simulink model "SimulinkModel"  (R2023a)
settings: Solver=FixedStepAuto  StartTime=0.0  StopTime=10  FixedStep=DT  RelTol=1e-3
values from neighbouring files (symbols this model uses):
  A = [0 1 0 0 ... (first row only)    [Main.m]
  AO = A-KO*C    [Main.m]
  B1 = [0; b12; 0; b14]    [Main.m]
  B2 = [0 0 0 0 ... (first row only)    [Main.m]
  BO = B1-KO*D1    [Main.m]
  C = [1 0 0 0 ... (first row only)    [Main.m]
  Ce = [ 1 0 0 0]    [Main.m]
  Ceps = [-ks/ms -bs/ms 0 0 0 ... (first row only)    [Main.m]
  CO = eye(n)    [Main.m]
  D1 = [0; 1/ms]    [Main.m]
  D2 = [0 1 0 0 ... (first row only)    [Main.m]
  De1 = 0    [Main.m]
  De2 = [0 0 1 -1]    [Main.m]
  Deps = [1/ms; 0; 0; 0;0; 0]    [Main.m]
  DT = 1e-3    (= 0.001)    [Main.m]
  e0 = x0(1)-r0    [Main.m]
  KI = K(:,n+1:n+m)    [Main.m]
  KO = Km.'    [Main.m]
  KS = K(:,1:n)    [Main.m]
  m = 1    [Main.m]
  n = size(V)    [JCF.m]    (also in Main.m = 4)
  p = 1    [Main.m]
  PLANT = 1    [Main.m]
  q = length(index{i})    [JCF.m]    (also in Main.m = 2)
  r = w(4)    [F.m]    (also in Main.m = 4; reference.m = 0.34671875)
  r0 = ells-g*ms/ks    (= 0.367749146758)    [Main.m]    (also in reference.m = 0.34671875)
  tilde_x_init = x_init-x0    [Main.m]
  u0 = 0    [Main.m]
  v = 10    [Main.m]
  w0 = [d0; nu0; r0]    [Main.m]
  x0 = [ells-g*ms/ks ... (first row only)    [Main.m]
  x_init = [zs_init-zu_init ... (first row only)    [Main.m]
  xO_init = tilde_x_init    [Main.m]
  y0 = [x0(1) ... (first row only)    [Main.m]
libraries: simulink x3
settings Model: Creator=nicola.mimmo2  LastModifiedBy=loreb
settings DebuggingCC: UnconnectedInputMsg=warning  UnconnectedOutputMsg=warning  UnconnectedLineMsg=warning
settings ModelReferenceCC: EnableRefExpFcnMdlSchedulingChecks=on
settings RTWCC: DLArmComputeVersion=19.05

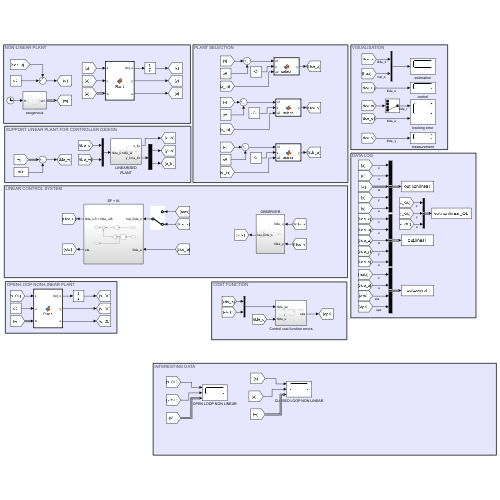
[thumbnail: Simulink's stored preview of the top-level diagram]
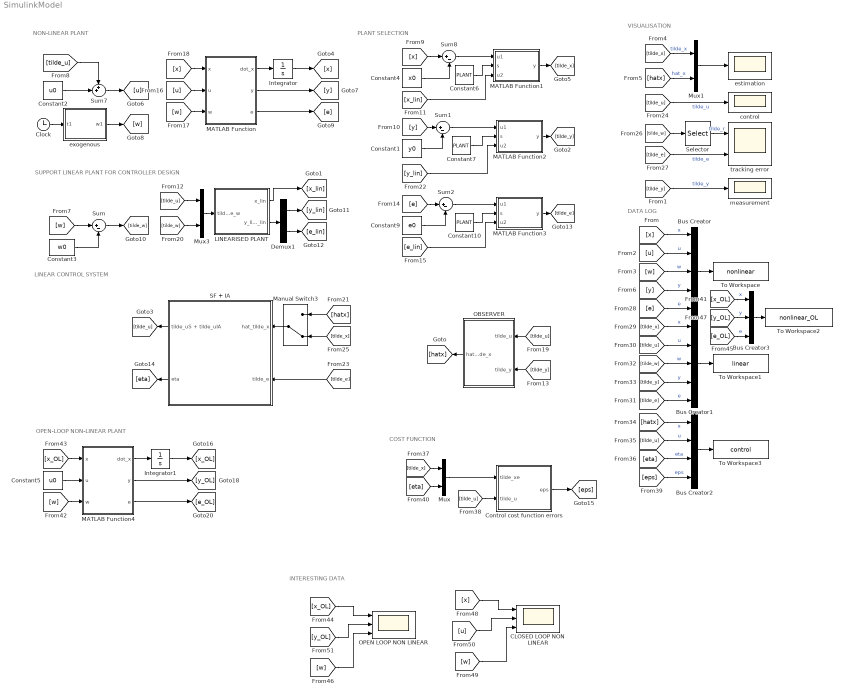
== system SimulinkModel ==
  note: DATA LOG
  note: VISUALISATION
  note: PLANT SELECTION
  note: NON-LINEAR PLANT
  note: SUPPORT LINEAR PLANT FOR CONTROLLER DESIGN
  note: LINEAR CONTROL SYSTEM
  note: OPEN-LOOP NON-LINEAR PLANT
  note: COST FUNCTION
  note: iNTERESTING DATA
  Bus Creator : BusCreator  Inputs=5
  Bus Creator1 : BusCreator  Inputs=5
  Bus Creator2 : BusCreator  Inputs=4
  Bus Creator3 : BusCreator  Inputs=3
  CLOSED LOOP NON LINEAR : Scope  NumInputPorts=3
  Clock : Clock
  Constant1 : Constant  Value=y0
  Constant10 : Constant  Value=PLANT
  Constant2 : Constant  Value=u0
  Constant3 : Constant  Value=w0
  Constant4 : Constant  Value=x0
  Constant5 : Constant  Value=u0
  Constant6 : Constant  Value=PLANT
  Constant7 : Constant  Value=PLANT
  Constant9 : Constant  Value=e0
  Control cost function errors : Subsystem
  Demux1 : Demux  Outputs=[q m]
  Integrator : Integrator  InitialCondition=x_init
  Integrator1 : Integrator  InitialCondition=x_init
  LINEARISED PLANT : Subsystem
  MATLAB Function : MATLAB Function  TreatAsAtomicUnit=on
  MATLAB Function1 : MATLAB Function  TreatAsAtomicUnit=on
  MATLAB Function2 : MATLAB Function  TreatAsAtomicUnit=on
  MATLAB Function3 : MATLAB Function  TreatAsAtomicUnit=on
  MATLAB Function4 : MATLAB Function  TreatAsAtomicUnit=on
  Manual Switch3 : ManualSwitch  CurrentSetting=0
  Mux : Mux  Inputs=2
  Mux1 : Mux  Inputs=2
  Mux3 : Mux  Inputs=2
  OBSERVER : Subsystem
  OPEN LOOP NON LINEAR : Scope  NumInputPorts=3
  SF + IA : Subsystem
  Selector : Selector  InputPortWidth=r  IndexOptions=Index vector (dialog)  Indices=[r-m+1:1:r]  OutputSizes=1
  Sum{,1..2,8} (4 alike) : Sum  Inputs=|+-
  Sum7 : Sum  Inputs=++|
  To Workspace : ToWorkspace  VariableName=nonlinear  SaveFormat=Timeseries  SampleTime=-1
  To Workspace1 : ToWorkspace  VariableName=linear  SaveFormat=Timeseries  SampleTime=-1
  To Workspace2 : ToWorkspace  VariableName=nonlinear_OL  SaveFormat=Timeseries  SampleTime=-1
  To Workspace3 : ToWorkspace  VariableName=control  SaveFormat=Timeseries  SampleTime=-1
  control : Scope
  estimation : Scope
  exogenous : Subsystem
  measurement : Scope
  tracking error : Scope  NumInputPorts=2
  wires:
  Integrator/1 -> [x]
  Constant3/1 -> Sum/2
  Mux3/1 -> LINEARISED PLANT/1(tilde_u tilde_w)
  OBSERVER/1(hat_tilde_x) -> [hatx]
  [tilde_x] -> Mux1/1  "tilde_x"
  [hatx] -> Mux1/2  "hat_x"
  SF + IA/1(tilde_uS + tilde_uIA) -> [tilde_u]
  Constant2/1 -> Sum7/2
  Sum7/1 -> [u]
  [tilde_u] -> Sum7/1
  Constant1/1 -> Sum1/2
  Sum1/1 -> MATLAB Function2/1(u1)
  [y] -> Sum1/1
  [w] -> Sum/1
  [x] -> Sum8/1
  Constant4/1 -> Sum8/2
  Sum8/1 -> MATLAB Function1/1(u1)
  [x_lin] -> MATLAB Function1/3(u2)
  [tilde_e] -> SF + IA/2(tilde_e)
  [tilde_u] -> Mux3/1
  [u] -> MATLAB Function/2(u)
  [w] -> MATLAB Function/3(w)
  [x] -> MATLAB Function/1(x)
  Sum/1 -> [tilde_w]
  [tilde_w] -> Mux3/2
  [y_lin] -> MATLAB Function2/3(u2)
  Demux1/1 -> [y_lin]
  Demux1/2 -> [e_lin]
  [tilde_u] -> OBSERVER/1(tilde_u)
  Manual Switch3/1 -> SF + IA/1(hat_tilde_x)
  [hatx] -> Manual Switch3/1
  [tilde_x] -> Manual Switch3/2
  MATLAB Function/3(e) -> [e]
  MATLAB Function/2(y) -> [y]
  LINEARISED PLANT/1(x_lin) -> [x_lin]
  LINEARISED PLANT/2(y_lin e_lin) -> Demux1/1
  Clock/1 -> exogenous/1(t1)
  exogenous/1(w1) -> [w]
  MATLAB Function/1(dot_x) -> Integrator/1
  Mux1/1 -> estimation/1
  Constant6/1 -> MATLAB Function1/2(s)
  MATLAB Function1/1(y) -> [tilde_x]
  Constant7/1 -> MATLAB Function2/2(s)
  [tilde_y] -> OBSERVER/2(tilde_y)
  [e_lin] -> MATLAB Function3/3(u2)
  Constant9/1 -> Sum2/2
  Sum2/1 -> MATLAB Function3/1(u1)
  Constant10/1 -> MATLAB Function3/2(s)
  [e] -> Sum2/1
  [tilde_u] -> control/1  "tilde_u"
  [tilde_w] -> Selector/1
  Selector/1 -> tracking error/1  "tilde_r"
  [tilde_e] -> tracking error/2  "tilde_e"
  [tilde_y] -> measurement/1  "tilde_y"
  [y] -> Bus Creator/4  "y"
  [e] -> Bus Creator/5  "e"
  [w] -> Bus Creator/3  "w"
  [u] -> Bus Creator/2  "u"
  [x] -> Bus Creator/1  "x"
  Bus Creator/1 -> To Workspace/1
  [tilde_u] -> Bus Creator1/2  "u"
  [tilde_w] -> Bus Creator1/3  "w"
  [tilde_x] -> Bus Creator1/1  "x"
  [tilde_e] -> Bus Creator1/5  "e"
  [tilde_y] -> Bus Creator1/4  "y"
  Bus Creator1/1 -> To Workspace1/1
  SF + IA/2(eta) -> [eta]
  MATLAB Function2/1(y) -> [tilde_y]
  MATLAB Function3/1(y) -> [tilde_e]
  [hatx] -> Bus Creator2/1  "x"
  [tilde_u] -> Bus Creator2/2  "u"
  [eta] -> Bus Creator2/3  "eta"
  Bus Creator2/1 -> To Workspace3/1
  [tilde_u] -> Control cost function errors/2(tilde_u)
  Control cost function errors/1(eps) -> [eps]
  [eps] -> Bus Creator2/4  "eps"
  [tilde_x] -> Mux/1
  [eta] -> Mux/2
  Mux/1 -> Control cost function errors/1(tilde_xe)
  Integrator1/1 -> [x_OL]
  MATLAB Function4/3(e) -> [e_OL]
  MATLAB Function4/2(y) -> [y_OL]
  Constant5/1 -> MATLAB Function4/2(u)
  MATLAB Function4/1(dot_x) -> Integrator1/1
  [x_OL] -> MATLAB Function4/1(x)
  [w] -> MATLAB Function4/3(w)
  Bus Creator3/1 -> To Workspace2/1
  [x_OL] -> Bus Creator3/1  "x"
  [y_OL] -> Bus Creator3/2  "y"
  [e_OL] -> Bus Creator3/3  "e"
  [x_OL] -> OPEN LOOP NON LINEAR/1
  [w] -> CLOSED LOOP NON LINEAR/3
  [x] -> CLOSED LOOP NON LINEAR/1
  [u] -> CLOSED LOOP NON LINEAR/2
  [y_OL] -> OPEN LOOP NON LINEAR/2
  [w] -> OPEN LOOP NON LINEAR/3

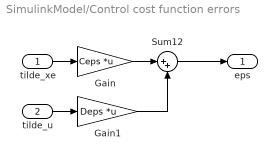
== system SimulinkModel/Control cost function errors ==
  tilde_xe : Inport
  tilde_u : Inport  Port=2
  Gain : Gain  Gain=Ceps  Multiplication=Matrix(K*u)
  Gain1 : Gain  Gain=Deps  Multiplication=Matrix(K*u)
  Sum12 : Sum  Inputs=|++
  eps : Outport
  wires:
  Gain1/1 -> Sum12/2
  Gain/1 -> Sum12/1
  Sum12/1 -> eps/1
  tilde_xe/1 -> Gain/1
  tilde_u/1 -> Gain1/1

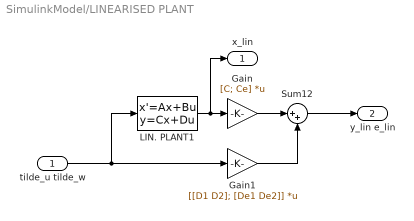
== system SimulinkModel/LINEARISED PLANT ==
  tilde_u tilde_w : Inport
  Gain : Gain  Gain=[C; Ce]  Multiplication=Matrix(K*u)
  Gain1 : Gain  Gain=[[D1 D2]; [De1 De2]]  Multiplication=Matrix(K*u)
  LIN. PLANT1 : StateSpace  A=A  B=[B1 B2]  C=eye(n)  D=zeros(n,p+r)  InitialCondition=tilde_x_init
  Sum12 : Sum  Inputs=|++
  x_lin : Outport
  y_lin e_lin : Outport  Port=2
  wires:
  Gain1/1 -> Sum12/2
  tilde_u tilde_w/1 -> Gain1/1, LIN. PLANT1/1
  Gain/1 -> Sum12/1
  LIN. PLANT1/1 -> x_lin/1, Gain/1
  Sum12/1 -> y_lin e_lin/1

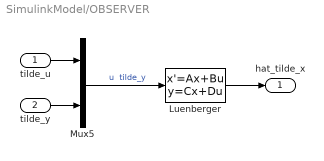
== system SimulinkModel/OBSERVER ==
  tilde_u : Inport
  tilde_y : Inport  Port=2
  Luenberger : StateSpace  A=AO  B=[BO KO]  C=CO  D=zeros(n,p+q)  InitialCondition=xO_init
  Mux5 : Mux  Inputs=2
  hat_tilde_x : Outport
  wires:
  tilde_u/1 -> Mux5/1
  Mux5/1 -> Luenberger/1  "u  tilde_y"
  tilde_y/1 -> Mux5/2
  Luenberger/1 -> hat_tilde_x/1

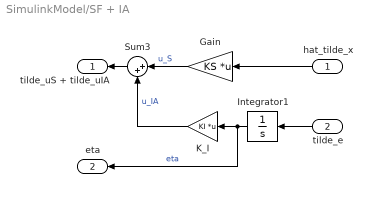
== system SimulinkModel/SF + IA ==
  hat_tilde_x : Inport
  tilde_e : Inport  Port=2
  Gain : Gain  Gain=KS  Multiplication=Matrix(K*u)
  Integrator1 : Integrator
  K_I : Gain  Gain=KI  Multiplication=Matrix(K*u)
  Sum3 : Sum  Inputs=|++
  tilde_uS + tilde_uIA : Outport
  eta : Outport  Port=2
  wires:
  Gain/1 -> Sum3/1  "u_S"
  Integrator1/1 -> eta/1, K_I/1  "eta"
  tilde_e/1 -> Integrator1/1
  K_I/1 -> Sum3/2  "u_IA"
  hat_tilde_x/1 -> Gain/1
  Sum3/1 -> tilde_uS + tilde_uIA/1

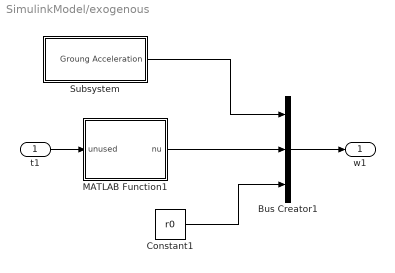
== system SimulinkModel/exogenous ==
  t1 : Inport
  Bus Creator1 : BusCreator  Inputs=3
  Constant1 : Constant  Value=r0
  MATLAB Function1 : MATLAB Function  TreatAsAtomicUnit=on  SystemSampleTime=DT
  Subsystem : Subsystem
  w1 : Outport
  wires:
  Constant1/1 -> Bus Creator1/3
  Bus Creator1/1 -> w1/1
  MATLAB Function1/1(nu) -> Bus Creator1/2
  t1/1 -> MATLAB Function1/1(unused)
  Subsystem/1(Groung Acceleration) -> Bus Creator1/1

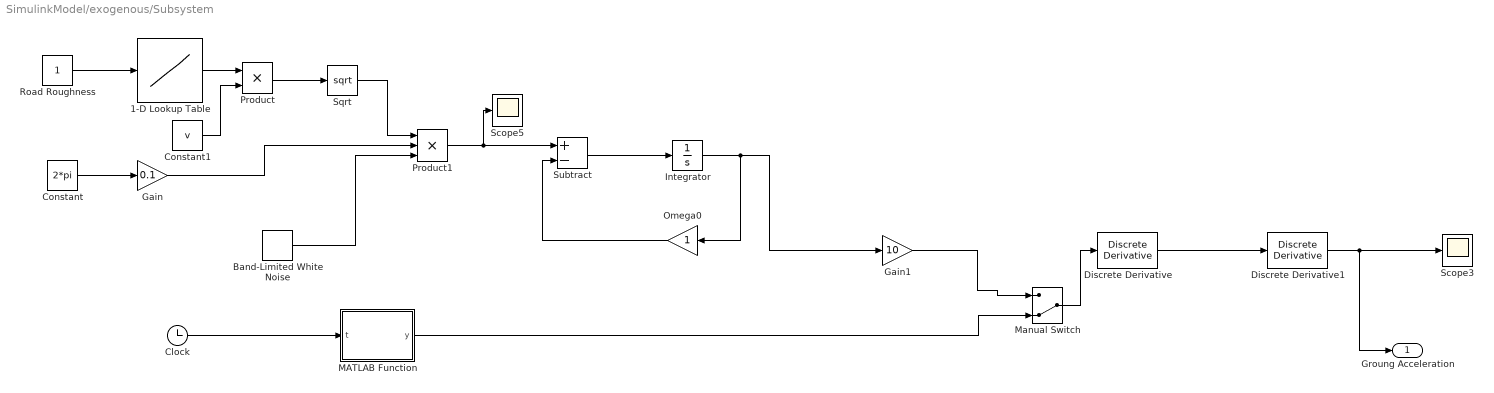
== system SimulinkModel/exogenous/Subsystem ==
  1-D Lookup Table : Lookup_n-D  NumberOfTableDimensions=1  BreakpointsForDimension1=[1;2;3;4;5;6;7;8]  Table=[1.6e-05;6.4e-05;0.000256;0.001024;0.004096;0.016384;0.065536;0.262144]  InternalRulePriority=Speed  RndMeth=Simplest
  Band-Limited White Noise : simulink/Sources/Band-Limited White Noise  Cov=0.1  Ts=0.01  seed=[23341]
  Clock : Clock
  Constant : Constant  Value=2*pi
  Constant1 : Constant  Value=v
  Discrete Derivative : simulink/Quick Insert/Discrete/Discrete Derivative  gainval=1.0  ICPrevScaledInput=0.0  OutMin=[]  OutMax=[]  OutDataType=fixdt(1, 16)  OutScaling=2^-10  DoSatur=off
  Discrete Derivative1 : simulink/Quick Insert/Discrete/Discrete Derivative  gainval=1.0  ICPrevScaledInput=0.0  OutMin=[]  OutMax=[]  OutDataType=fixdt(1, 16)  OutScaling=2^-10  DoSatur=off
  Gain : Gain  Gain=0.1
  Gain1 : Gain  Gain=10
  Integrator : Integrator
  MATLAB Function : MATLAB Function  TreatAsAtomicUnit=on
  Manual Switch : ManualSwitch  CurrentSetting=0
  Omega0 : Gain
  Product : Product
  Product1 : Product  Inputs=3
  Road Roughness : Constant
  Scope3 : Scope
  Scope5 : Scope
  Sqrt : Sqrt
  Subtract : Sum  Inputs=+-
  Groung Acceleration : Outport
  wires:
  Subtract/1 -> Integrator/1
  Road Roughness/1 -> 1-D Lookup Table/1
  Clock/1 -> MATLAB Function/1(t)
  1-D Lookup Table/1 -> Product/1
  Sqrt/1 -> Product1/1
  Constant/1 -> Gain/1
  Band-Limited White Noise/1 -> Product1/3
  Omega0/1 -> Subtract/2
  MATLAB Function/1(y) -> Manual Switch/2
  Product1/1 -> Scope5/1, Subtract/1
  Integrator/1 -> Omega0/1, Gain1/1
  Constant1/1 -> Product/2
  Product/1 -> Sqrt/1
  Gain/1 -> Product1/2
  ? -> ?
  Gain1/1 -> Manual Switch/1
  Discrete Derivative/1 -> Discrete Derivative1/1
  Discrete Derivative1/1 -> Groung Acceleration/1, Scope3/1
  Manual Switch/1 -> Discrete Derivative/1

== matlab function SimulinkModel/MATLAB Function1 ==
  data: u1 input; s input; y output; u2 input
function y = select(u1,s,u2)

if s == 0
    y = u2;
else
    y = u1;
end

== matlab function SimulinkModel/MATLAB Function ==
  data: x input; u input; dot_x output; w input; y output; e output
function [dot_x,y,e] = Plant(x,u,w)
[dot_x,y,e] = F(x,u,w);
end

== matlab function SimulinkModel/MATLAB Function2 ==
  data: u1 input; s input; y output; u2 input
function y = select(u1,s,u2)

if s == 0
    y = u2;
else
    y = u1;
end

== matlab function SimulinkModel/MATLAB Function3 ==
  data: u1 input; s input; y output; u2 input
function y = select(u1,s,u2)

if s == 0
    y = u2;
else
    y = u1;
end

== matlab function SimulinkModel/MATLAB Function4 ==
  data: x input; u input; dot_x output; w input; y output; e output
function [dot_x,y,e] = Plant(x,u,w)
[dot_x,y,e] = F(x,u,w);
end

== matlab function SimulinkModel/exogenous/MATLAB Function1 ==
  data: unused input; nu output
function nu = noises(~)
std_pot = 0.001; % [m] potentiomenter standard deviation
std_acc = 110e-6*sqrt(200); % [m/s^2] accelerometer standard deviation
nu = [std_pot*(2*rand(1)-1)
      std_acc*(2*rand(1)-1)];

end

== matlab function SimulinkModel/exogenous/Subsystem/MATLAB Function ==
  data: t input; y output
function y = fcn(t)

% Parameters definition

v = 10; % [m/s] speed of the vehicle

p = v*t; % [m] position that varies with time

pg = 20; % [m] pg is the position of the BEGINNING of the bump

l = 1; % [m] lenght of the hole/bump
h = 0.2; % [m] thickness of the hole/bump

lmat = [l^4 l^5 l^6 l^7 l^8; (l/2)^4 (l/2)^5 (l/2)^6 (l/2)^7 (l/2)^8; 4*l^3 5*l^4 6*l^5 7*l^6 8*l^7; 12*l^2 20*l^3 30*l^4 42*l^5 56*l^6; 24*l 60*l^2 120*l^3 210*l^4 336*l^5;];
lmatinv = inv(lmat);

cmat = zeros(5,1);
hmat = [0 h 0 0 0]';

cmat = lmatinv * hmat;

% Road profile function

if (p>pg && p-pg < l)
    sum = 0;
    for i = 0:8
        if i > 3
            sum = sum + cmat(i-3)*(p-pg)^(i);
        end
    end
    y = sum;
else
    y = 0;
end
